simulink model "Traffic_lights_R202a0"  (R2020a)
settings: Solver=FixedStepAuto  StartTime=0.0  StopTime=10.0  MaxStep=1e-3  RelTol=1e-3  EnableMultiTasking=on
libraries: arduinolib x5, dspswit3 x3
settings Model: SILPILModeSetting=veronly  ExtModeTrigDuration=2  Creator=hp  LastModifiedBy=hp
settings OptimizationCC: EnhancedBackFolding=on  PassReuseOutputArgsAs=Individual arguments  ZeroExternalMemoryAtStartup=off  ZeroInternalMemoryAtStartup=off  MaxStackSize=64  OptimizeBlockOrder=speed  DifferentSizesBufferReuse=on  OptimizationCustomize=off  EfficientTunableParamExpr=on
settings DebuggingCC: ParameterTunabilityLossMsg=error  UnconnectedInputMsg=none  UnconnectedOutputMsg=none  UnconnectedLineMsg=none
settings HardwareCC: ProdBitPerInt=16  ProdBitPerPointer=16  ProdBitPerSizeT=16  ProdBitPerPtrDiffT=16  ProdLargestAtomicFloat=None  ProdWordSize=8  ProdHWDeviceType=Atmel->AVR
settings ModelReferenceCC: EnableRefExpFcnMdlSchedulingChecks=off
settings SFSimCC: MATLABDynamicMemAlloc=off
settings RTWCC: SystemTargetFile=ert.tlc  HardwareBoard=Arduino Uno  TLCOptions=-aInlineSetEventsForThisBaseRateFcn=TLC_FALSE -aSuppressMultiTaskScheduler=TLC_FALSE -aRateBasedStepFcn=1  TemplateMakefile=ert_default_tmf  Toolchain=Arduino AVR  BuildConfiguration=Faster Runs
settings CodeAppCC: ForceParamTrailComments=on  IgnoreCustomStorageClasses=off  OperatorAnnotations=on  SimulinkDataObjDesc=on  SFDataObjDesc=on  InsertBlockDesc=on
settings ERTTargetCC: SupportContinuousTime=on  SupportVariableSizeSignals=on  ExtModeTransport=3  ExtModeStaticAlloc=on  ExtModeStaticAllocSize=250  ExtModeMexFile=ext_xcp  ExtModeIntrfLevel=Level2 - Open

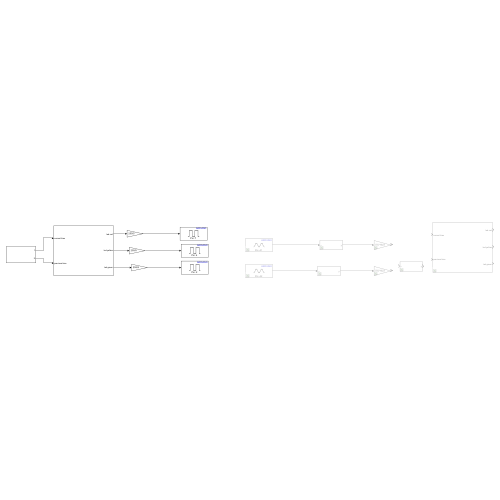
[thumbnail: Simulink's stored preview of the top-level diagram]
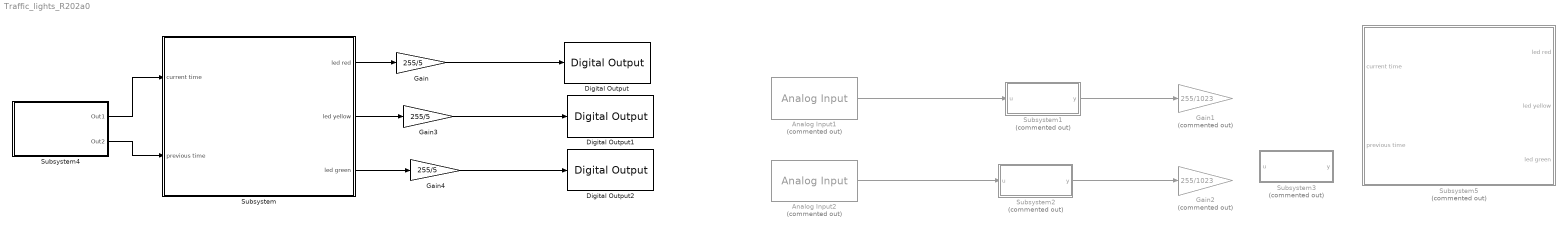
== system Traffic_lights_R202a0 ==
  Analog Input1 : arduinolib/Analog Input  Commented=on  pinNumber=1  ReadResultsOnly=off  ConversionTriggerSource=Software  ExternalTriggerType=uint32( 0 )  OutputDataType=uint16  EnableConversionCompleteNotify=off  EnableOuputStatus=off  SampleTime=-1  blockPlatform=arduino
  Analog Input2 : arduinolib/Analog Input  Commented=on  pinNumber=2  ReadResultsOnly=off  ConversionTriggerSource=Software  ExternalTriggerType=uint32( 0 )  OutputDataType=uint16  EnableConversionCompleteNotify=off  EnableOuputStatus=off  SampleTime=-1  blockPlatform=arduino
  Digital Output : arduinolib/Digital Output  pinNumber=7  Direction=output  blockPlatform=arduino
  Digital Output1 : arduinolib/Digital Output  pinNumber=4  Direction=output  blockPlatform=arduino
  Digital Output2 : arduinolib/Digital Output  pinNumber=2  Direction=output  blockPlatform=arduino
  Gain : Gain  Gain=255/5
  Gain1 : Gain  Commented=on  Gain=255/1023
  Gain2 : Gain  Commented=on  Gain=255/1023
  Gain3 : Gain  Gain=255/5
  Gain4 : Gain  Gain=255/5
  Subsystem : Subsystem
  Subsystem1 : Subsystem  Commented=on
  Subsystem2 : Subsystem  Commented=on
  Subsystem3 : Subsystem  Commented=on
  Subsystem4 : Subsystem
  Subsystem5 : Subsystem  Commented=on
  wires:
  Analog Input1/1 -> Subsystem1/1(u)
  Subsystem1/1(y) -> Gain1/1
  Analog Input2/1 -> Subsystem2/1(u)
  Subsystem2/1(y) -> Gain2/1
  Subsystem/1(led red) -> Gain/1
  Gain/1 -> Digital Output/1
  Subsystem/3(led green) -> Gain4/1
  Gain4/1 -> Digital Output2/1
  Gain3/1 -> Digital Output1/1
  Subsystem/2(led yellow) -> Gain3/1
  Subsystem4/1(Out1) -> Subsystem/1(current time)
  Subsystem4/2(Out2) -> Subsystem/2(previous time)

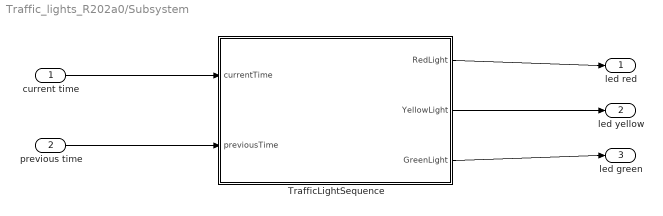
== system Traffic_lights_R202a0/Subsystem ==
  current time : Inport
  previous time : Inport  Port=2
  TrafficLightSequence : MATLAB Function  TreatAsAtomicUnit=on
  led red : Outport
  led yellow : Outport  Port=2
  led green : Outport  Port=3
  wires:
  current time/1 -> TrafficLightSequence/1(currentTime)
  previous time/1 -> TrafficLightSequence/2(previousTime)
  TrafficLightSequence/1(RedLight) -> led red/1
  TrafficLightSequence/2(YellowLight) -> led yellow/1
  TrafficLightSequence/3(GreenLight) -> led green/1

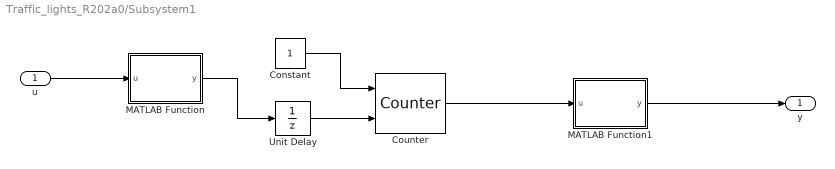
== system Traffic_lights_R202a0/Subsystem1 ==
  u : Inport
  Constant : Constant
  Counter : dspswit3/Counter  Direction=Up  CountEvent=Rising edge  CounterSize=User defined  MaxCount=255  InitialCount=0  Output=Count  HitValue=32  ResetInput=on  SamplesPerFrame=1  Ts=1  CntDtype=double  HitDtype=Logical
  MATLAB Function : MATLAB Function  TreatAsAtomicUnit=on
  MATLAB Function1 : MATLAB Function  TreatAsAtomicUnit=on
  Unit Delay : UnitDelay  SampleTime=-1  HasFrameUpgradeWarning=on
  y : Outport
  wires:
  Constant/1 -> Counter/1
  MATLAB Function1/1(y) -> y/1
  Counter/1 -> MATLAB Function1/1(u)
  MATLAB Function/1(y) -> Unit Delay/1
  u/1 -> MATLAB Function/1(u)
  Unit Delay/1 -> Counter/2

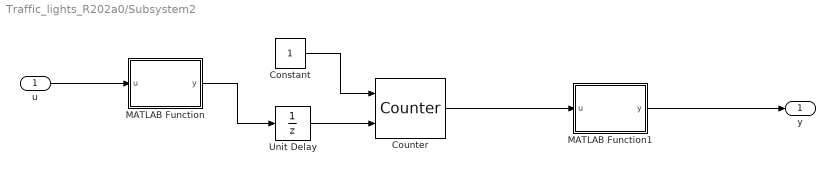
== system Traffic_lights_R202a0/Subsystem2 ==
  u : Inport
  Constant : Constant
  Counter : dspswit3/Counter  Direction=Up  CountEvent=Rising edge  CounterSize=User defined  MaxCount=255  InitialCount=0  Output=Count  HitValue=32  ResetInput=on  SamplesPerFrame=1  Ts=1  CntDtype=double  HitDtype=Logical
  MATLAB Function : MATLAB Function  TreatAsAtomicUnit=on
  MATLAB Function1 : MATLAB Function  TreatAsAtomicUnit=on
  Unit Delay : UnitDelay  SampleTime=-1  HasFrameUpgradeWarning=on
  y : Outport
  wires:
  Unit Delay/1 -> Counter/2
  u/1 -> MATLAB Function/1(u)
  MATLAB Function/1(y) -> Unit Delay/1
  Counter/1 -> MATLAB Function1/1(u)
  MATLAB Function1/1(y) -> y/1
  Constant/1 -> Counter/1

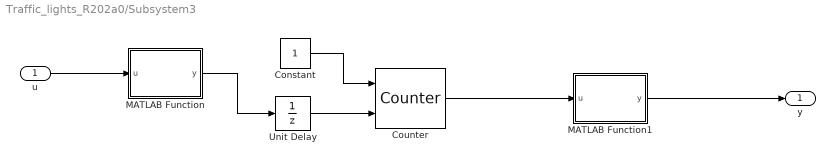
== system Traffic_lights_R202a0/Subsystem3 ==
  u : Inport
  Constant : Constant
  Counter : dspswit3/Counter  Direction=Up  CountEvent=Rising edge  CounterSize=User defined  MaxCount=255  InitialCount=0  Output=Count  HitValue=32  ResetInput=on  SamplesPerFrame=1  Ts=1  CntDtype=double  HitDtype=Logical
  MATLAB Function : MATLAB Function  TreatAsAtomicUnit=on
  MATLAB Function1 : MATLAB Function  TreatAsAtomicUnit=on
  Unit Delay : UnitDelay  SampleTime=0.5  HasFrameUpgradeWarning=on
  y : Outport
  wires:
  Constant/1 -> Counter/1
  MATLAB Function1/1(y) -> y/1
  Counter/1 -> MATLAB Function1/1(u)
  MATLAB Function/1(y) -> Unit Delay/1
  u/1 -> MATLAB Function/1(u)
  Unit Delay/1 -> Counter/2

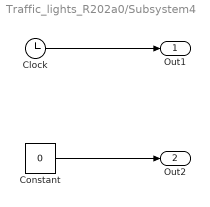
== system Traffic_lights_R202a0/Subsystem4 ==
  Clock : Clock
  Constant : Constant  Value=0
  Out1 : Outport
  Out2 : Outport  Port=2
  wires:
  Constant/1 -> Out2/1
  Clock/1 -> Out1/1

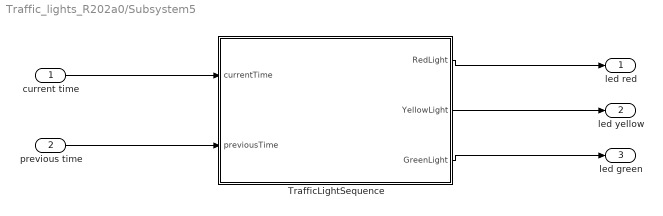
== system Traffic_lights_R202a0/Subsystem5 ==
  current time : Inport
  previous time : Inport  Port=2
  TrafficLightSequence : MATLAB Function  TreatAsAtomicUnit=on
  led red : Outport
  led yellow : Outport  Port=2
  led green : Outport  Port=3
  wires:
  TrafficLightSequence/3(GreenLight) -> led green/1
  TrafficLightSequence/2(YellowLight) -> led yellow/1
  TrafficLightSequence/1(RedLight) -> led red/1
  previous time/1 -> TrafficLightSequence/2(previousTime)
  current time/1 -> TrafficLightSequence/1(currentTime)

== matlab function Traffic_lights_R202a0/Subsystem5/TrafficLightSequence ==
  data: currentTime input; RedLight output; previousTime input; YellowLight output; GreenLight output
function [RedLight, YellowLight, GreenLight] = TrafficLightSequence(currentTime, previousTime)
    % Traffic light sequence with delays
    
    % Define timing parameters (in seconds)
    redTime = 10;
    yellowTime = 5;
    greenTime = 11;

    % Initialize outputs
    RedLight = 0;
    YellowLight = 0;
    GreenLight = 0;

    % Calculate elapsed time since the last update
    elapsedTime = currentTime - previousTime;

    % Traffic light sequence logic
    if elapsedTime >= redTime + yellowTime + greenTime
        % Reset the timer
        previousTime = currentTime;
    end

    if elapsedTime < redTime
        % Red light is ON
        RedLight = 1;
    elseif elapsedTime < redTime + yellowTime
        % Yellow light is ON
        YellowLight = 1;
    else
        % Green light is ON
        GreenLight = 1;
    end
end

== matlab function Traffic_lights_R202a0/Subsystem/TrafficLightSequence ==
  data: currentTime input; RedLight output; previousTime input; YellowLight output; GreenLight output
function [RedLight, YellowLight, GreenLight] = TrafficLightSequenceContinuous(currentTime, previousTime)
    % Continuous traffic light sequence
    
    % Adjust timing parameters (in seconds)
    redTime = 5;     % Set the duration for the red light
    yellowTime =5;   % Set the duration for the yellow light
    greenTime = 5;   % Set the duration for the green light

    % Initialize outputs
    RedLight = 0;
    YellowLight = 0;
    GreenLight = 0;

    % Calculate elapsed time since the last update
    elapsedTime = currentTime - previousTime;

    % Calculate the time within a complete cycle
    cycleTime = redTime + yellowTime + greenTime;

    % Determine the current phase in the cycle
    currentPhase = mod(elapsedTime, cycleTime);

    % Traffic light sequence logic
    if currentPhase < redTime
        % Red light is ON
        RedLight = 1;
    elseif currentPhase < redTime + yellowTime
        % Yellow light is ON
        YellowLight = 1;
    else
        % Green light is ON
        GreenLight = 1;
    end
end

== matlab function Traffic_lights_R202a0/Subsystem1/MATLAB Function ==
  data: u input; y output
function y = fcn(u)
If u ==6
y=1;
Else
y=0;
end

== matlab function Traffic_lights_R202a0/Subsystem1/MATLAB Function1 ==
  data: u input; y output
function y = fcn(u)

if u == 0
    Led red = 0;
    Led yellow =1;
    Led Green = 0;
    
end

== matlab function Traffic_lights_R202a0/Subsystem2/MATLAB Function ==
  data: u input; y output
function y = fcn(u)
If u ==9
y=1;
Else
y=0;
end

== matlab function Traffic_lights_R202a0/Subsystem2/MATLAB Function1 ==
  data: u input; y output
function y = fcn(u)

if u == 0
    Led red = 0;
    Led yellow = 0;
    Led Green =1;
    
end

== matlab function Traffic_lights_R202a0/Subsystem3/MATLAB Function ==
  data: u input; y output
function y = fcn(u)
If u ==3
y=1;
Else
y=0;
end

== matlab function Traffic_lights_R202a0/Subsystem3/MATLAB Function1 ==
  data: u input; y output
function y = fcn(u)

if u == 0
    Led red = 1;
    Led yellow = 0;
    Led Green = 0;
elseif
 Led red = 0;
    Led yellow = 1;
    Led Green = 0;
else
    Led red = 0;
    Led yellow = 0;
    Led Green = 1;
    
end
